simulink model "PTtest"  (R2021a)
settings: Solver=VariableStepAuto  StartTime=0.0  StopTime=3  RelTol=1e-3
undefined symbols (not defined in the file or in its folder): National_Instruments, PCIe
libraries: sldrtlib x7
settings Model: Creator=simmo536  LastModifiedBy=simmo536

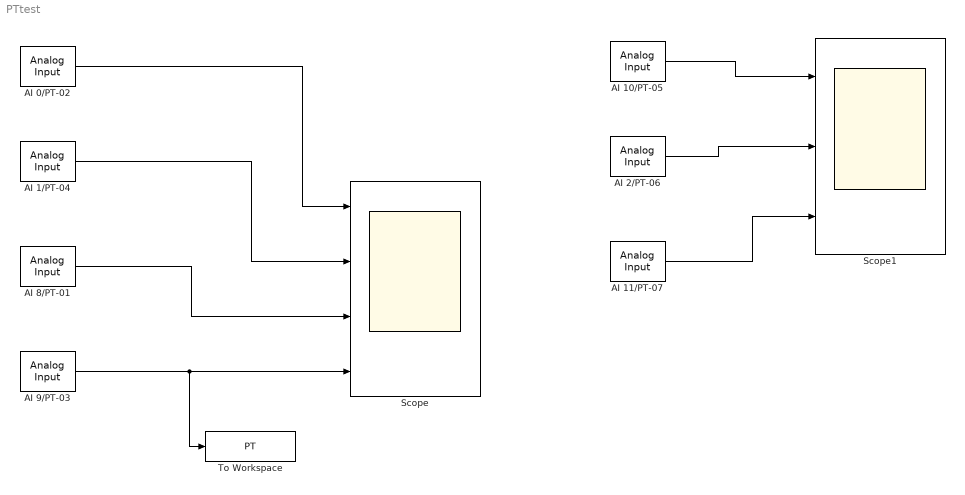
== system PTtest ==
  AI 0/PT-02 : sldrtlib/Analog Input  SampleTime=0.01  MaxMissedTicks=inf  ShowMissedTicks=off  YieldWhenWaiting=on  DrvName=National_Instruments/PCIe-6343  DrvAddress=4294967295  DrvOptions=[0 0 0 0 0 0 0]  Channels=1  RangeMode=1  VoltRange=1  DataType=2
      settings: AttributesFormatString=National Instruments\nPCIe-6343 [auto]
  AI 1/PT-04 : sldrtlib/Analog Input  SampleTime=0.01  MaxMissedTicks=inf  ShowMissedTicks=off  YieldWhenWaiting=off  DrvName=National_Instruments/PCIe-6343  DrvAddress=4294967295  DrvOptions=[0 0 0 0 0 0 0]  Channels=2  RangeMode=1  VoltRange=1  DataType=2
      settings: AttributesFormatString=National Instruments\nPCIe-6343 [auto]
  AI 10/PT-05 : sldrtlib/Analog Input  SampleTime=0.01  MaxMissedTicks=inf  ShowMissedTicks=off  YieldWhenWaiting=on  DrvName=National_Instruments/PCIe-6343  DrvAddress=4294967295  DrvOptions=[0 0 0 0 0 0 0]  Channels=11  RangeMode=1  VoltRange=1  DataType=2
      settings: AttributesFormatString=National Instruments\nPCIe-6343 [auto]
  AI 11/PT-07 : sldrtlib/Analog Input  SampleTime=0.01  MaxMissedTicks=inf  ShowMissedTicks=off  YieldWhenWaiting=on  DrvName=National_Instruments/PCIe-6343  DrvAddress=4294967295  DrvOptions=[0 0 0 0 0 0 0]  Channels=12  RangeMode=1  VoltRange=1  DataType=2
      settings: AttributesFormatString=National Instruments\nPCIe-6343 [auto]
  AI 2/PT-06 : sldrtlib/Analog Input  SampleTime=0.01  MaxMissedTicks=inf  ShowMissedTicks=off  YieldWhenWaiting=off  DrvName=National_Instruments/PCIe-6343  DrvAddress=4294967295  DrvOptions=[0 0 0 0 0 0 0]  Channels=3  RangeMode=1  VoltRange=1  DataType=2
      settings: AttributesFormatString=National Instruments\nPCIe-6343 [auto]
  AI 8/PT-01 : sldrtlib/Analog Input  SampleTime=0.01  MaxMissedTicks=inf  ShowMissedTicks=off  YieldWhenWaiting=on  DrvName=National_Instruments/PCIe-6343  DrvAddress=4294967295  DrvOptions=[0 0 0 0 0 0 0]  Channels=16  RangeMode=1  VoltRange=1  DataType=2
      settings: AttributesFormatString=National Instruments\nPCIe-6343 [auto]
  AI 9/PT-03 : sldrtlib/Analog Input  SampleTime=0.01  MaxMissedTicks=inf  ShowMissedTicks=off  YieldWhenWaiting=off  DrvName=National_Instruments/PCIe-6343  DrvAddress=4294967295  DrvOptions=[0 0 0 0 0 0 0]  Channels=10  RangeMode=1  VoltRange=1  DataType=2
      settings: AttributesFormatString=National Instruments\nPCIe-6343 [auto]
  Scope : Scope  NumInputPorts=4
  Scope1 : Scope  NumInputPorts=3
  To Workspace : ToWorkspace  VariableName=PT  SaveFormat=Timeseries  SampleTime=-1
  wires:
  AI 0/PT-02/1 -> Scope/1
  AI 1/PT-04/1 -> Scope/2
  AI 8/PT-01/1 -> Scope/3
  AI 9/PT-03/1 -> To Workspace/1, Scope/4
  AI 11/PT-07/1 -> Scope1/3
  AI 2/PT-06/1 -> Scope1/2
  AI 10/PT-05/1 -> Scope1/1
